simulink model "circuit"  (R2018a)
settings: Solver=VariableStepAuto  StartTime=0.0  StopTime=sim_time  FixedStep=sim_step  RelTol=1e-3
values from neighbouring files (symbols this model uses):
  den = [1 0]    [optimPID.m]    (also in run.m = [1 1])
  kp = 14.98    [run.m]
  num = [1]    [run.m]
  T = 0.01    [run.m]
  tau = 0.1    [run.m]
  Td = 4.343    [run.m]
  Ti = 1.592    [run.m]
settings Model: Creator=barthap  LastModifiedBy=barthap

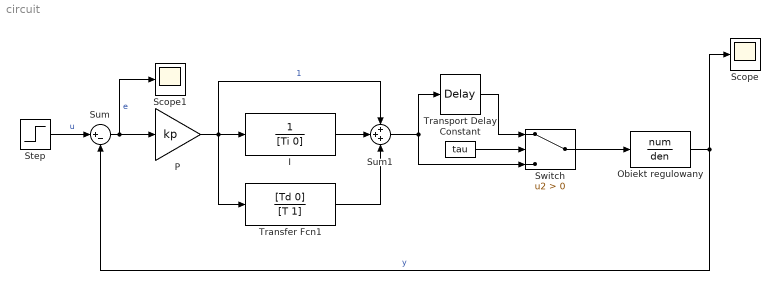
== system circuit ==
  Constant : Constant  Value=tau
  I : TransferFcn  Denominator=[Ti 0]
  Obiekt regulowany : TransferFcn  Numerator=num  Denominator=den
  P : Gain  Gain=kp
  Scope : Scope
  Scope1 : Scope
  Step : Step  Time=0  SampleTime=0
  Sum : Sum  Inputs=|+-
  Sum1 : Sum  Inputs=+++
  Switch : Switch  Criteria=u2 > Threshold
  Transfer Fcn1 : TransferFcn  Numerator=[Td 0]  Denominator=[T 1]
  Transport Delay : TransportDelay  DelayTime=tau
  wires:
  Step/1 -> Sum/1  "u"
  Sum/1 -> Scope1/1, P/1  "e"
  P/1 -> Sum1/1, I/1, Transfer Fcn1/1  "1"
  I/1 -> Sum1/2
  Transfer Fcn1/1 -> Sum1/3
  Obiekt regulowany/1 -> Scope/1, Sum/2  "y"
  Constant/1 -> Switch/2
  Sum1/1 -> Transport Delay/1, Switch/3
  Transport Delay/1 -> Switch/1
  Switch/1 -> Obiekt regulowany/1
